simulink model "untitled"  (R2021b)
settings: Solver=VariableStepAuto  StartTime=0.0  StopTime=10.0  RelTol=1e-3
settings Model: Creator=K Yasaswini  LastModifiedBy=K Yasaswini

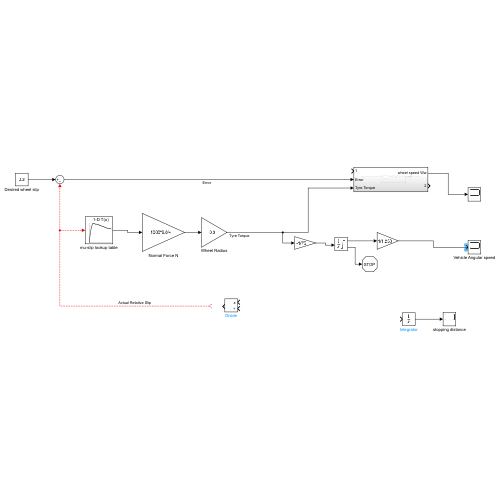
[thumbnail: Simulink's stored preview of the top-level diagram]
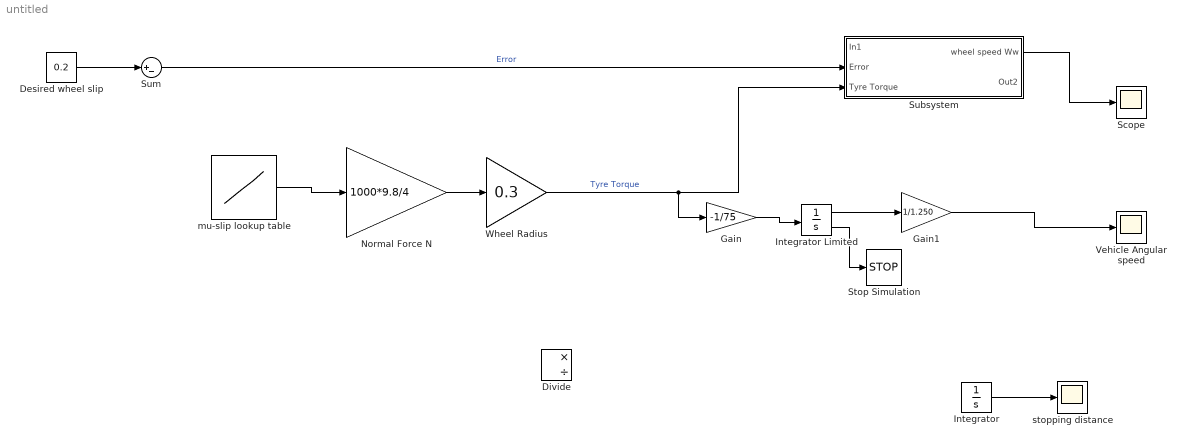
== system untitled ==
  Desired wheel slip : Constant  Value=0.2
  Divide : Product  Inputs=*/
  Gain : Gain  Gain=-1/75
  Gain1 : Gain  Gain=1/1.250
  Integrator : Integrator
  Integrator Limited : Integrator  InitialCondition=44  LimitOutput=on  UpperSaturationLimit=1000  LowerSaturationLimit=0  ShowSaturationPort=on
  Normal Force N : Gain  Gain=1000*9.8/4
  Scope : Scope
  Stop Simulation : Stop
  Subsystem : Subsystem
  Sum : Sum  Inputs=|+-
  Vehicle Angular speed : Scope
  Wheel Radius : Gain  Gain=0.3
  mu-slip lookup table : Lookup_n-D  NumberOfTableDimensions=1  BreakpointsForDimension1=[0,0.05,0.1,0.15,0.2,0.25,0.3,0.35,0.4,0.45,0.5,0.55,0.6,0.65,0.7,0.75,0.8,0.85,0.9,0.95,1]  Table=[0,0.4,0.8,0.97,1,0.98,0.96,0.94,0.92,0.9,0.88,0.855,0.83,0.81,0.79,0.77,0.75,0.73,0.72,0.71,0.7]  InternalRulePriority=Speed  RndMeth=Simplest  InputSameDT=on
  stopping distance : Scope
  wires:
  Desired wheel slip/1 -> Sum/1
  ? -> Sum/2, mu-slip lookup table/1  "Actual Relative Slip"
  mu-slip lookup table/1 -> Normal Force N/1
  Normal Force N/1 -> Wheel Radius/1
  Sum/1 -> Subsystem/2(Error)  "Error"
  Wheel Radius/1 -> Gain/1, Subsystem/3(Tyre Torque)  "Tyre Torque"
  Subsystem/1(wheel speed Ww) -> Scope/1
  Gain/1 -> Integrator Limited/1
  Integrator Limited/1 -> Gain1/1
  Integrator Limited/2 -> Stop Simulation/1
  Integrator/1 -> stopping distance/1
  Gain1/1 -> Vehicle Angular speed/1

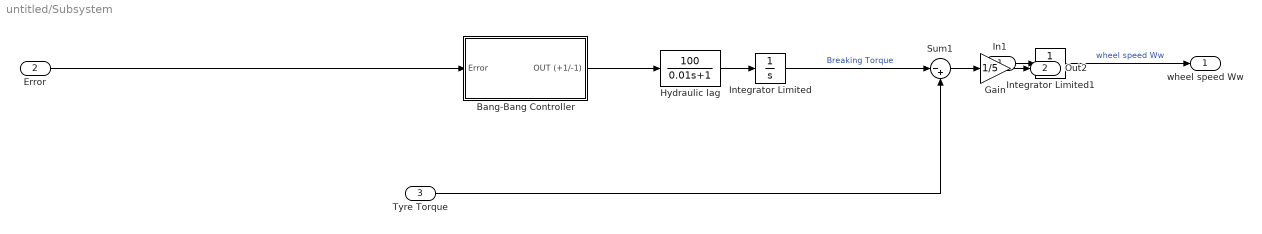
== system untitled/Subsystem ==
  In1 : Inport
  Error : Inport  Port=2
  Tyre Torque : Inport  Port=3
  Bang-Bang Controller : Subsystem
  Gain : Gain  Gain=1/5
  Hydraulic lag : TransferFcn  Numerator=[100]  Denominator=[0.01 1]
  Integrator Limited : Integrator  LimitOutput=on  UpperSaturationLimit=1000  LowerSaturationLimit=0
  Integrator Limited1 : Integrator  InitialCondition=44/1.2500  LimitOutput=on  UpperSaturationLimit=1000  LowerSaturationLimit=0
  Sum1 : Sum  Inputs=|-+
  wheel speed Ww : Outport
  Out2 : Outport  Port=2
  wires:
  Gain/1 -> Out2/1
  Tyre Torque/1 -> Sum1/2
  Integrator Limited/1 -> Sum1/1  "Breaking Torque"
  Hydraulic lag/1 -> Integrator Limited/1
  Bang-Bang Controller/1(OUT (+1/-1)) -> Hydraulic lag/1
  Integrator Limited1/1 -> wheel speed Ww/1  "wheel speed Ww"
  Error/1 -> Bang-Bang Controller/1(Error)
  Sum1/1 -> Gain/1
  In1/1 -> Integrator Limited1/1

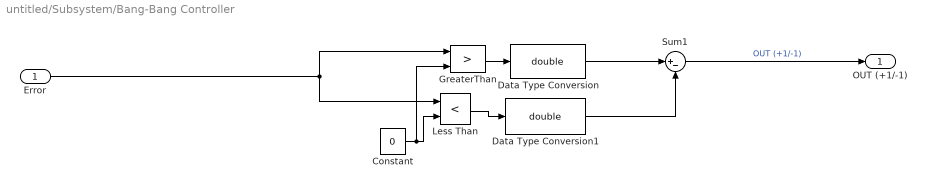
== system untitled/Subsystem/Bang-Bang Controller ==
  Error : Inport
  Constant : Constant  Value=0
  Data Type Conversion : DataTypeConversion  OutDataTypeStr=double  RndMeth=Zero
  Data Type Conversion1 : DataTypeConversion  OutDataTypeStr=double  RndMeth=Zero
  GreaterThan : RelationalOperator  Operator=>  OutDataTypeStr=boolean  RndMeth=Simplest
  Less Than : RelationalOperator  Operator=<  OutDataTypeStr=boolean  RndMeth=Simplest
  Sum1 : Sum  Inputs=|+-
  OUT (+1/-1) : Outport
  wires:
  GreaterThan/1 -> Data Type Conversion/1
  Error/1 -> GreaterThan/1, Less Than/1
  Sum1/1 -> OUT (+1/-1)/1  "OUT (+1/-1)"
  Data Type Conversion/1 -> Sum1/1
  Data Type Conversion1/1 -> Sum1/2
  Constant/1 -> GreaterThan/2, Less Than/2
  Less Than/1 -> Data Type Conversion1/1
